simulink library "ADRC_Toolbox"  (R2024a)
settings: Solver=VariableStepAuto  StartTime=0.0  StopTime=10.0  RelTol=1e-3
undefined symbols (not defined in the file or in its folder): build_robot_screw, ToolGroup, ToolSet, Ts, x0
libraries: $bdroot x14, simulink x7
(part 2 of 2)

== matlab function ADRC_Toolbox/Advanced Motor Control/TD/order3_LTD/set matrix ==
  data: freq input size=1; A output; B output; C output; D output
function [A,B,C,D] = fcn(freq)
N = 3; % 阶数
wc = 2*pi*freq;
w = wc / sqrt(2^(1/N) - 1); 
A = zeros(N,N);
for k = 1:N-1
    A(k, k+1) = 1;
end
for k = 1:N
    A(N, k) = -nchoosek(N,k-1) * w^(N-k+1) ;
end
B = zeros(N,1);
B(N) = w^N;
C = zeros(3,N);
C(1,1) = 1;
C(2,2) = 1;
C(3,3) = 1;
D = 0;
end

== matlab function ADRC_Toolbox/Advanced Motor Control/TD/order3_LTD/set x0 ==
  data: u input double size=1; x0 output double
function x0 = set_x0(u)
N = 3; %阶数
x0 = zeros(N,1);
x0(1) = u;

== matlab function ADRC_Toolbox/Interface/encoder2physical_PC ==
  data: PC_encoder input Bus: Arm_Bus size=1; PC_physical output Bus: Arm_Bus size=1
function PC_physical  = e2p_PC(PC_encoder)

PC_physical = encoder2physical_PC(PC_encoder);
end

== matlab function ADRC_Toolbox/Advanced Motor Control/TD/order5_LTD /set matrix ==
  data: freq input size=1; A output; B output; C output; D output
function [A,B,C,D] = fcn(freq)
N = 5; % 阶数
wc = 2*pi*freq;
w = wc / sqrt(2^(1/N) - 1); 
A = zeros(N,N);
for k = 1:N-1
    A(k, k+1) = 1;
end
for k = 1:N
    A(N, k) = -nchoosek(N,k-1) * w^(N-k+1) ;
end
B = zeros(N,1);
B(N) = w^N;
C = zeros(3,N);
C(1,1) = 1;
C(2,2) = 1;
C(3,3) = 1;
D = 0;
end

== matlab function ADRC_Toolbox/Advanced Motor Control/TD/order2_LTD/set matrix ==
  data: freq input size=1; A output; B output; C output; D output
function [A,B,C,D] = fcn(freq)
N = 2; % 阶数
wc = 2*pi*freq;
w = wc / sqrt(2^(1/N) - 1); 
A = zeros(N,N);
for k = 1:N-1
    A(k, k+1) = 1;
end
for k = 1:N
    A(N, k) = -nchoosek(N,k-1) * w^(N-k+1) ;
end
B = zeros(N,1);
B(N) = w^N;
C = eye(2);
D = 0;
end

== matlab function ADRC_Toolbox/Advanced Motor Control/TD/order2_LTD/set x0 ==
  data: u input double size=1; x0 output double
function x0 = set_x0(u)
N = 2; %阶数
x0 = zeros(N,1);
x0(1) = u;

== matlab function ADRC_Toolbox/Advanced Motor Control/TD/order2_LTD with speed limit/MATLAB Function ==
  data: x input; u output; v input; freq input
function u = fcn(x, v, freq)
N = 2;
wc = 2*pi*freq;
w = wc / sqrt(2^(1/N) - 1); 

u = -w^2 * x(1) - 2*w*x(2) + w^2*v;

== matlab function ADRC_Toolbox/Advanced Motor Control/TD/order2_LTD with speed limit/MATLAB Function2 ==
  data: x input; y output; alpha input; v input
function y = fcn(x, alpha, v)

y = alpha.*(v - x(2));

== matlab function ADRC_Toolbox/Advanced Motor Control/TD/order2_LTD with speed limit/set matrix ==
  data: A output; B output; C output; D output
function [A,B,C,D] = fcn()
A = [0 1; 0 0];
B = [0 ; 1];
C = eye(2);
D = 0;
end

== matlab function ADRC_Toolbox/Advanced Motor Control/TD/order2_LTD with speed limit/set x0 ==
  data: u input double size=1; x0 output double
function x0 = set_x0(u)
N = 2; %阶数
x0 = zeros(N,1);
x0(1) = u;

== matlab function ADRC_Toolbox/Advanced Motor Control/TD/order2_LTD with speed acc limit/MATLAB Function ==
  data: x input; u output; v input; freq input
function u = fcn(x, v, freq)
N = 2;
wc = 2*pi*freq;
w = wc / sqrt(2^(1/N) - 1); 

u = -w^2 * x(1) - 2*w*x(2) + w^2*v;

== matlab function ADRC_Toolbox/Interface/physical2encoder_PC ==
  data: PC_physical input Bus: Arm_Bus size=1; PC_encoder output Bus: Arm_Bus size=1
function PC_encoder  = p2e_PC(PC_physical)
PC_encoder = physical2encoder_PC(PC_physical);

end

== matlab function ADRC_Toolbox/Advanced Motor Control/TD/order2_LTD with speed acc limit/MATLAB Function2 ==
  data: x input; y output; alpha input; v input
function y = fcn(x, alpha, v)

y = alpha.*(v - x(2));

== matlab function ADRC_Toolbox/Advanced Motor Control/TD/order2_LTD with speed acc limit/set matrix ==
  data: A output; B output; C output; D output
function [A,B,C,D] = fcn()
A = [0 1; 0 0];
B = [0 ; 1];
C = eye(2);
D = 0;
end

== matlab function ADRC_Toolbox/Advanced Motor Control/TD/order2_LTD with speed acc limit/set x0 ==
  data: u input double size=1; x0 output double
function x0 = set_x0(u)
N = 2; %阶数
x0 = zeros(N,1);
x0(1) = u;

== matlab function ADRC_Toolbox/Advanced Motor Control/TD/order5_LTD /set x0 ==
  data: u input double size=1; x0 output double
function x0 = set_x0(u)
N = 5; %阶数
x0 = zeros(N,1);
x0(1) = u;

== matlab function ADRC_Toolbox/Advanced Motor Control/TD/order7_LTD/set matrix ==
  data: freq input size=1; A output; B output; C output; D output
function [A,B,C,D] = fcn(freq)
N = 7; % 阶数
wc = 2*pi*freq;
w = wc / sqrt(2^(1/N) - 1); 
A = zeros(N,N);
for k = 1:N-1
    A(k, k+1) = 1;
end
for k = 1:N
    A(N, k) = -nchoosek(N,k-1) * w^(N-k+1) ;
end
B = zeros(N,1);
B(N) = w^N;
C = zeros(3,N);
C(1,1) = 1;
C(2,2) = 1;
C(3,3) = 1;
D = 0;
end

== matlab function ADRC_Toolbox/Advanced Motor Control/TD/order7_LTD/set x0 ==
  data: u input double size=1; x0 output double
function x0 = set_x0(u)
N = 7; %阶数
x0 = zeros(N,1);
x0(1) = u;

== matlab function ADRC_Toolbox/Advanced Motor Control/TD/order9_LTD/set matrix ==
  data: freq input size=1; A output; B output; C output; D output
function [A,B,C,D] = fcn(freq)
N = 9; % 阶数
wc = 2*pi*freq;
w = wc / sqrt(2^(1/N) - 1); 
A = zeros(N,N);
for k = 1:N-1
    A(k, k+1) = 1;
end
for k = 1:N
    A(N, k) = -nchoosek(N,k-1) * w^(N-k+1) ;
end
B = zeros(N,1);
B(N) = w^N;
C = zeros(3,N);
C(1,1) = 1;
C(2,2) = 1;
C(3,3) = 1;
D = 0;
end

== matlab function ADRC_Toolbox/Advanced Motor Control/TD/order9_LTD/set x0 ==
  data: u input double size=1; x0 output double
function x0 = set_x0(u)
N = 9; %阶数
x0 = zeros(N,1);
x0(1) = u;

== matlab function ADRC_Toolbox/tools/Stapler Tmatrix ==
  data: theta_motor input size=14; T output size=[4,4]; P input Bus: Config_Stapler_Bus size=1; open output size=1
function [T, open] = Stapler_T(theta_motor, P)
% body = theta_motor(1:5);
arm = theta_motor(6:9);
MD = theta_motor(10:14);

screw = build_Stapler(P);
[theta_joint, open] = screw.MDMotor2EndTool(arm, MD);

T = screw.FK(theta_joint);

end

== matlab function ADRC_Toolbox/Advanced Motor Control/Controller/LADRC 2nd/1//b1 ==
  data: u input; out output; b0 input
function out = b0(u, b0)
epsi = 1e-8;
if b0 < epsi
    out = 0;
else
    out = u/b0;
end

== matlab function ADRC_Toolbox/Advanced Motor Control/Controller/LADRC 2nd/MATLAB Function ==
  data: y input; x0 output
function x0 = init(y)
x0 = [y; 0; 0];
end

== matlab function ADRC_Toolbox/Advanced Motor Control/Controller/LADRC 2nd/MATLAB Function1 ==
  data: wo input; A output; b0 input; B output; C output; D output
function [A, B, C, D] = fcn(wo, b0)
A = [-3*wo 1 0;-3*wo^2 0 1;-wo^3 0 0];
B = [0 3*wo;b0 3*wo^2 ; 0 wo^3 ];
C = eye(3);
D = zeros(3,2);

== matlab function ADRC_Toolbox/Advanced Motor Control/Controller/LADRC 2nd/derr_Kd1 ==
  data: u input; out output; wc input
function out = kd(u, wc)

out = u * wc * 2;

== matlab function ADRC_Toolbox/Advanced Motor Control/Controller/LADRC 2nd/err_Kp1 ==
  data: u input; out output; wc input
function out = kp(u, wc)

out = u * wc^2;

== matlab function ADRC_Toolbox/tools/NormalTool_T2 ==
  data: theta_motor input size=14; T output size=[4,4]; P input Bus: Config_NormalTool2_Bus size=1; open output size=1
function [T, open] = NormalTool_T2(theta_motor, P)
% body = theta_motor(1:5);
arm = theta_motor(6:9);
MD = theta_motor(10:14);

screw = build_NormalTool2(P);
[theta_joint, open] = screw.MDMotor2EndTool(arm, MD);

T = screw.FK(theta_joint);
end

== matlab function ADRC_Toolbox/tools/Screenangle2T ==
  data: screen_angle input; Tscreen output
function Tscreen = screenangle2T(screen_angle)
theta = screen_angle/180*pi;
R = [0 0 1;
     0 1 0;
     -1 0 0];
p = [0;0;0];
M = [R,p;[0 0 0 1]];
s = [0; -1; 0; 0; 0; 0];
Tscreen = expm(VecTose3(s)*theta) * M;
end

== matlab function ADRC_Toolbox/Interface/allocateAllHands ==
  data: SC1 output Bus: Hand_Bus size=1; SC2 output Bus: Hand_Bus size=1; SC3 output Bus: Hand_Bus size=1; SC4 output Bus: Hand_Bus size=1; SC_L input Bus: Hand_Bus size=1; SC_R input Bus: Hand_Bus size=1; ErrorCode output double size=1
function [SC1, SC2, SC3, SC4, ErrorCode] = allocateAllHands(SC_L, SC_R)

%% 分配index  左手1 右手2
SC_L.index = uint16(1);
SC_R.index = uint16(2);

%% 根据臂号复制
[index, ErrorCode] = SC_allocate(SC_L.matching_index, SC_R.matching_index);
SC0 = empty_SC();
SCs = {SC0,SC0,SC0,SC0};

for k = 1:4
    switch index(k)
        case 1
            SCs{k} = SC_L;
        case 2
            SCs{k} = SC_R;
        otherwise
    end
end

SC1 = SCs{1};
SC2 = SCs{2};
SC3 = SCs{3};
SC4 = SCs{4};
end

== stateflow chart ADRC_Toolbox/utils/Error Merge/Error Merge ==
  state checkerror
    du:
    ErrorMemery = ErrorCode;
  state wait
    en:
    ErrorMemery = ErrorCode;
  (default) -> wait
  wait -> checkerror : [ErrorCode > 0]
  checkerror -> wait : [ErrorCode == 0]
  data: ErrorCode input uint16 size=1; ErrorMemery data_store_memory

== matlab function ADRC_Toolbox/utils/Tform2Vec/Tform2Vec ==
  data: T input; eul_angle output; p output
function [eul_angle, p] = Tform2Vec(T)
% 将位姿矩阵转为位移和欧拉角
p = T(1:3, 4);
eul = tform2eul(T);
eul_angle = eul * 180 / pi;

== matlab function ADRC_Toolbox/Interface/SC PC concat/checkToolType ==
  data: tooltype input size=1; flag output size=1; ErrorCode output size=1
function [flag, ErrorCode] = checkToolType(tooltype)
[flag, ErrorCode] = isToolTypeValid(tooltype);
end

== matlab function ADRC_Toolbox/Interface/SC PC concat/isScope ==
  data: tooltype input; flag output
function flag = isScope(tooltype)
flag = isEndscope(tooltype);
end
